simulink model "eVTOL_System"  (R2024b)
settings: Solver=FixedStepAuto  StartTime=0.0  StopTime=inf  RelTol=1e-3
undefined symbols (not defined in the file): airspeed, Battery, BCE12, BCE_Set_init, BMS_Controller_State, C, Cell10_P, Cell11_P, Cell12_P, Cell13_P, Cell14_P, Cell15_P, Cell16_P, Cell17_P, Cell18_P, Cell19_P, Cell1_N, Cell1_P, Cell20_P, Cell21_P, Cell22_P, Cell23_P, Cell24_P, Cell2_P, Cell3_P, Cell4_P, Cell5_P, Cell6_P, Cell7_P, Cell8_P, Cell9_P, Charging_State, CityMission, control, controlParams, ControlSampleTime, CriticalTiltAngle, currentFactor, CV_Gain, ddx, ddy, ddz, Device_01, Device_02, DiscIntNeverNeededParam, dx, dy, dz, Earth, env, F, F28379D_ADC_MaxCount, F28379D_ADC_Vmax, FixedWingMission, flightState, Foc_Ki_IxTcpu, Foc_Ki_S, Foc_Kp_I, Foc_Kp_S, fractalcoef ... (+68)
libraries: fl_lib x1115, nesl_utility x617, slrealtimeethercatlib x217, simulink x130, canmsglib x101, speedgoatlib_IO611_obsolete x91, slpidlib x49, mcbcontrolslib x44, slrealtimeutilitieslib x35, speedgoatlib_hdlCoder_IO3xx x31, dspstat3 x24, mcbpositiondecoderlib x12
(part 27 of 31)

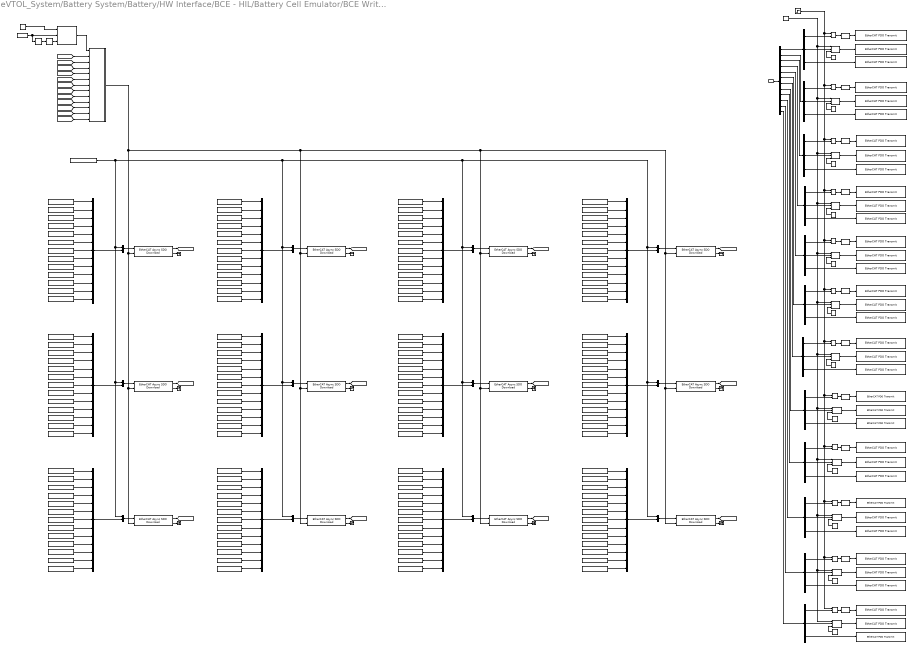
== system eVTOL_System/Battery System/Battery/HW Interface/BCE - HIL/Battery Cell Emulator/BCE Write 1/Subsystem/BCE Write  ==
  note: Task Scheduling
  note: Cell 4
  note: Cell 5
  note: Setup
  note: Cell 8
  note: Cell 8
  note: Cell 9
  note: Cell 1
  note: Cell 7
  note: Update
  note: Cell 2
  note: Cell 10
  note: Cell 1
  note: Cell 5
  note: Cell 3
  note: Cell 11
  note: Cell 10
  note: Cell 6
  note: Cell 7
  note: Cell 12
  note: Cell 6
  note: Cell 9
  note: Cell 11
  note: Cell 3
  note: Cell 12
  note: Cell 4
  note: Cell 2
  Data : Inport  OutDataTypeStr=Bus: BCE_Set
  BceVoltageLimit : Constant  Value=5  SampleTime=0.001
  Bus Selector : BusSelector  OutputSignals=Cell_1,Cell_2,Cell_3,Cell_4,Cell_5,Cell_6,Cell_7,Cell_8,Cell_9,Cell_10,Cell_11,Cell_12
  Bus Selector{1..12} (12 alike) : BusSelector  OutputSignals=Enable,V,I
  CellEnableDelay : Step  Time=2  SampleTime=0.001
  Constant{,1..11} (12 alike) : Constant  Value=0
  Data Type Conversion{1..12} (12 alike) : DataTypeConversion  OutDataTypeStr=uint8  SaturateOnIntegerOverflow=off  RndMeth=Floor
  Enable until confirmed : Subsystem
  EtherCAT Async SDO Download01 : slrealtimeethercatlib/EtherCAT Async SDO Download  index=0x4001  subIndex=1  sig_type=uint16  sig_dim=14  device_id=0  subdevice_name=Device_02 (BCE12-0505)  sample_time=0.001  subdevice_addr=1002  selected_subdevice=BCE_01  timeout=500  subdevice_found=0  complete=1
  EtherCAT Async SDO Download02 : slrealtimeethercatlib/EtherCAT Async SDO Download  index=0x4002  subIndex=1  sig_type=uint16  sig_dim=14  device_id=0  subdevice_name=Device_02 (BCE12-0505)  sample_time=0.001  subdevice_addr=1002  selected_subdevice=BCE_01  timeout=500  subdevice_found=0  complete=1
  EtherCAT Async SDO Download03 : slrealtimeethercatlib/EtherCAT Async SDO Download  index=0x4003  subIndex=1  sig_type=uint16  sig_dim=14  device_id=0  subdevice_name=Device_02 (BCE12-0505)  sample_time=0.001  subdevice_addr=1002  selected_subdevice=BCE_01  timeout=500  subdevice_found=0  complete=1
  EtherCAT Async SDO Download04 : slrealtimeethercatlib/EtherCAT Async SDO Download  index=0x4004  subIndex=1  sig_type=uint16  sig_dim=14  device_id=0  subdevice_name=Device_02 (BCE12-0505)  sample_time=0.001  subdevice_addr=1002  selected_subdevice=BCE_01  timeout=500  subdevice_found=0  complete=1
  EtherCAT Async SDO Download05 : slrealtimeethercatlib/EtherCAT Async SDO Download  index=0x4005  subIndex=1  sig_type=uint16  sig_dim=14  device_id=0  subdevice_name=Device_02 (BCE12-0505)  sample_time=0.001  subdevice_addr=1002  selected_subdevice=BCE_01  timeout=500  subdevice_found=0  complete=1
  EtherCAT Async SDO Download06 : slrealtimeethercatlib/EtherCAT Async SDO Download  index=0x4006  subIndex=1  sig_type=uint16  sig_dim=14  device_id=0  subdevice_name=Device_02 (BCE12-0505)  sample_time=0.001  subdevice_addr=1002  selected_subdevice=BCE_01  timeout=500  subdevice_found=0  complete=1
  EtherCAT Async SDO Download07 : slrealtimeethercatlib/EtherCAT Async SDO Download  index=0x4007  subIndex=0  sig_type=uint16  sig_dim=14  device_id=0  subdevice_name=Device_02 (BCE12-0505)  sample_time=0.001  subdevice_addr=1002  selected_subdevice=BCE_01  timeout=500  subdevice_found=0  complete=1
  EtherCAT Async SDO Download08 : slrealtimeethercatlib/EtherCAT Async SDO Download  index=0x4008  subIndex=0  sig_type=uint16  sig_dim=14  device_id=0  subdevice_name=Device_02 (BCE12-0505)  sample_time=0.001  subdevice_addr=1002  selected_subdevice=BCE_01  timeout=500  subdevice_found=0  complete=1
  EtherCAT Async SDO Download09 : slrealtimeethercatlib/EtherCAT Async SDO Download  index=0x4009  subIndex=1  sig_type=uint16  sig_dim=14  device_id=0  subdevice_name=Device_02 (BCE12-0505)  sample_time=0.001  subdevice_addr=1002  selected_subdevice=BCE_01  timeout=500  subdevice_found=0  complete=1
  EtherCAT Async SDO Download10 : slrealtimeethercatlib/EtherCAT Async SDO Download  index=0x400A  subIndex=1  sig_type=uint16  sig_dim=14  device_id=0  subdevice_name=Device_02 (BCE12-0505)  sample_time=0.001  subdevice_addr=1002  selected_subdevice=BCE_01  timeout=500  subdevice_found=0  complete=1
  EtherCAT Async SDO Download11 : slrealtimeethercatlib/EtherCAT Async SDO Download  index=0x400B  subIndex=1  sig_type=uint16  sig_dim=14  device_id=0  subdevice_name=Device_02 (BCE12-0505)  sample_time=0.001  subdevice_addr=1002  selected_subdevice=BCE_01  timeout=500  subdevice_found=0  complete=1
  EtherCAT Async SDO Download12 : slrealtimeethercatlib/EtherCAT Async SDO Download  index=0x400C  subIndex=1  sig_type=uint16  sig_dim=14  device_id=0  subdevice_name=Device_02 (BCE12-0505)  sample_time=0.001  subdevice_addr=1002  selected_subdevice=BCE_01  timeout=500  subdevice_found=0  complete=1
  EtherCAT PDO Transmit01 : slrealtimeethercatlib/EtherCAT PDO Transmit  Priority=3  sig_name=Device_02 (BCE12-0505).Rx_Cell_01.setVoltage  sig_offset=872  sig_type=single  type_size=32  sig_dim=1  device_id=0  sample_time=0.001000
  EtherCAT PDO Transmit02 : slrealtimeethercatlib/EtherCAT PDO Transmit  Priority=3  sig_name=Device_02 (BCE12-0505).Rx_Cell_01.setCurrent  sig_offset=904  sig_type=single  type_size=32  sig_dim=1  device_id=0  sample_time=0.001000
  EtherCAT PDO Transmit03 : slrealtimeethercatlib/EtherCAT PDO Transmit  Priority=3  sig_name=Device_02 (BCE12-0505).Rx_Cell_02.setVoltage  sig_offset=944  sig_type=single  type_size=32  sig_dim=1  device_id=0  sample_time=0.001000
  EtherCAT PDO Transmit04 : slrealtimeethercatlib/EtherCAT PDO Transmit  Priority=3  sig_name=Device_02 (BCE12-0505).Rx_Cell_02.setCurrent  sig_offset=976  sig_type=single  type_size=32  sig_dim=1  device_id=0  sample_time=0.001000
  EtherCAT PDO Transmit05 : slrealtimeethercatlib/EtherCAT PDO Transmit  Priority=3  sig_name=Device_02 (BCE12-0505).Rx_Cell_03.setVoltage  sig_offset=1016  sig_type=single  type_size=32  sig_dim=1  device_id=0  sample_time=0.001000
  EtherCAT PDO Transmit06 : slrealtimeethercatlib/EtherCAT PDO Transmit  Priority=3  sig_name=Device_02 (BCE12-0505).Rx_Cell_03.setCurrent  sig_offset=1048  sig_type=single  type_size=32  sig_dim=1  device_id=0  sample_time=0.001000
  EtherCAT PDO Transmit07 : slrealtimeethercatlib/EtherCAT PDO Transmit  Priority=3  sig_name=Device_02 (BCE12-0505).Rx_Cell_04.setVoltage  sig_offset=1088  sig_type=single  type_size=32  sig_dim=1  device_id=0  sample_time=0.001000
  EtherCAT PDO Transmit08 : slrealtimeethercatlib/EtherCAT PDO Transmit  Priority=3  sig_name=Device_02 (BCE12-0505).Rx_Cell_04.setCurrent  sig_offset=1120  sig_type=single  type_size=32  sig_dim=1  device_id=0  sample_time=0.001000
  EtherCAT PDO Transmit09 : slrealtimeethercatlib/EtherCAT PDO Transmit  Priority=3  sig_name=Device_02 (BCE12-0505).Rx_Cell_05.setVoltage  sig_offset=1160  sig_type=single  type_size=32  sig_dim=1  device_id=0  sample_time=0.001000
  EtherCAT PDO Transmit1 : slrealtimeethercatlib/EtherCAT PDO Transmit  Priority=3  sig_name=Device_02 (BCE12-0505).Rx_Cell_01.enableCell  sig_offset=864  sig_type=uint8  type_size=8  sig_dim=1  device_id=0  sample_time=0.001000
  EtherCAT PDO Transmit10 : slrealtimeethercatlib/EtherCAT PDO Transmit  Priority=3  sig_name=Device_02 (BCE12-0505).Rx_Cell_05.setCurrent  sig_offset=1192  sig_type=single  type_size=32  sig_dim=1  device_id=0  sample_time=0.001000
  EtherCAT PDO Transmit11 : slrealtimeethercatlib/EtherCAT PDO Transmit  Priority=3  sig_name=Device_02 (BCE12-0505).Rx_Cell_06.setVoltage  sig_offset=1232  sig_type=single  type_size=32  sig_dim=1  device_id=0  sample_time=0.001000
  EtherCAT PDO Transmit12 : slrealtimeethercatlib/EtherCAT PDO Transmit  Priority=3  sig_name=Device_02 (BCE12-0505).Rx_Cell_06.setCurrent  sig_offset=1264  sig_type=single  type_size=32  sig_dim=1  device_id=0  sample_time=0.001000
  EtherCAT PDO Transmit13 : slrealtimeethercatlib/EtherCAT PDO Transmit  Priority=3  sig_name=Device_02 (BCE12-0505).Rx_Cell_07.setVoltage  sig_offset=1304  sig_type=single  type_size=32  sig_dim=1  device_id=0  sample_time=0.001000
  EtherCAT PDO Transmit14 : slrealtimeethercatlib/EtherCAT PDO Transmit  Priority=3  sig_name=Device_02 (BCE12-0505).Rx_Cell_07.setCurrent  sig_offset=1336  sig_type=single  type_size=32  sig_dim=1  device_id=0  sample_time=0.001000
  EtherCAT PDO Transmit15 : slrealtimeethercatlib/EtherCAT PDO Transmit  Priority=3  sig_name=Device_02 (BCE12-0505).Rx_Cell_08.setVoltage  sig_offset=1376  sig_type=single  type_size=32  sig_dim=1  device_id=0  sample_time=0.001000
  EtherCAT PDO Transmit16 : slrealtimeethercatlib/EtherCAT PDO Transmit  Priority=3  sig_name=Device_02 (BCE12-0505).Rx_Cell_08.setCurrent  sig_offset=1408  sig_type=single  type_size=32  sig_dim=1  device_id=0  sample_time=0.001000
  EtherCAT PDO Transmit17 : slrealtimeethercatlib/EtherCAT PDO Transmit  Priority=3  sig_name=Device_02 (BCE12-0505).Rx_Cell_09.setVoltage  sig_offset=1448  sig_type=single  type_size=32  sig_dim=1  device_id=0  sample_time=0.001000
  EtherCAT PDO Transmit18 : slrealtimeethercatlib/EtherCAT PDO Transmit  Priority=3  sig_name=Device_02 (BCE12-0505).Rx_Cell_09.setCurrent  sig_offset=1480  sig_type=single  type_size=32  sig_dim=1  device_id=0  sample_time=0.001000
  EtherCAT PDO Transmit19 : slrealtimeethercatlib/EtherCAT PDO Transmit  Priority=3  sig_name=Device_02 (BCE12-0505).Rx_Cell_10.setVoltage  sig_offset=1520  sig_type=single  type_size=32  sig_dim=1  device_id=0  sample_time=0.001000
  EtherCAT PDO Transmit2 : slrealtimeethercatlib/EtherCAT PDO Transmit  Priority=3  sig_name=Device_02 (BCE12-0505).Rx_Cell_02.enableCell  sig_offset=936  sig_type=uint8  type_size=8  sig_dim=1  device_id=0  sample_time=0.001000
  EtherCAT PDO Transmit20 : slrealtimeethercatlib/EtherCAT PDO Transmit  Priority=3  sig_name=Device_02 (BCE12-0505).Rx_Cell_10.setCurrent  sig_offset=1552  sig_type=single  type_size=32  sig_dim=1  device_id=0  sample_time=0.001000
  EtherCAT PDO Transmit21 : slrealtimeethercatlib/EtherCAT PDO Transmit  Priority=3  sig_name=Device_02 (BCE12-0505).Rx_Cell_11.setVoltage  sig_offset=1592  sig_type=single  type_size=32  sig_dim=1  device_id=0  sample_time=0.001000
  EtherCAT PDO Transmit22 : slrealtimeethercatlib/EtherCAT PDO Transmit  Priority=3  sig_name=Device_02 (BCE12-0505).Rx_Cell_11.setCurrent  sig_offset=1624  sig_type=single  type_size=32  sig_dim=1  device_id=0  sample_time=0.001000
  EtherCAT PDO Transmit23 : slrealtimeethercatlib/EtherCAT PDO Transmit  Priority=3  sig_name=Device_02 (BCE12-0505).Rx_Cell_12.setVoltage  sig_offset=1664  sig_type=single  type_size=32  sig_dim=1  device_id=0  sample_time=0.001000
  EtherCAT PDO Transmit24 : slrealtimeethercatlib/EtherCAT PDO Transmit  Priority=3  sig_name=Device_02 (BCE12-0505).Rx_Cell_12.setCurrent  sig_offset=1696  sig_type=single  type_size=32  sig_dim=1  device_id=0  sample_time=0.001000
  EtherCAT PDO Transmit25 : slrealtimeethercatlib/EtherCAT PDO Transmit  Priority=3  sig_name=Device_02 (BCE12-0505).Rx_Cell_10.enableCell  sig_offset=1512  sig_type=uint8  type_size=8  sig_dim=1  device_id=0  sample_time=0.001000
  EtherCAT PDO Transmit26 : slrealtimeethercatlib/EtherCAT PDO Transmit  Priority=3  sig_name=Device_02 (BCE12-0505).Rx_Cell_11.enableCell  sig_offset=1584  sig_type=uint8  type_size=8  sig_dim=1  device_id=0  sample_time=0.001000
  EtherCAT PDO Transmit27 : slrealtimeethercatlib/EtherCAT PDO Transmit  Priority=3  sig_name=Device_02 (BCE12-0505).Rx_Cell_12.enableCell  sig_offset=1656  sig_type=uint8  type_size=8  sig_dim=1  device_id=0  sample_time=0.001000
  EtherCAT PDO Transmit3 : slrealtimeethercatlib/EtherCAT PDO Transmit  Priority=3  sig_name=Device_02 (BCE12-0505).Rx_Cell_03.enableCell  sig_offset=1008  sig_type=uint8  type_size=8  sig_dim=1  device_id=0  sample_time=0.001000
  EtherCAT PDO Transmit4 : slrealtimeethercatlib/EtherCAT PDO Transmit  Priority=3  sig_name=Device_02 (BCE12-0505).Rx_Cell_04.enableCell  sig_offset=1080  sig_type=uint8  type_size=8  sig_dim=1  device_id=0  sample_time=0.001000
  EtherCAT PDO Transmit5 : slrealtimeethercatlib/EtherCAT PDO Transmit  Priority=3  sig_name=Device_02 (BCE12-0505).Rx_Cell_05.enableCell  sig_offset=1152  sig_type=uint8  type_size=8  sig_dim=1  device_id=0  sample_time=0.001000
  EtherCAT PDO Transmit6 : slrealtimeethercatlib/EtherCAT PDO Transmit  Priority=3  sig_name=Device_02 (BCE12-0505).Rx_Cell_06.enableCell  sig_offset=1224  sig_type=uint8  type_size=8  sig_dim=1  device_id=0  sample_time=0.001000
  EtherCAT PDO Transmit7 : slrealtimeethercatlib/EtherCAT PDO Transmit  Priority=3  sig_name=Device_02 (BCE12-0505).Rx_Cell_07.enableCell  sig_offset=1296  sig_type=uint8  type_size=8  sig_dim=1  device_id=0  sample_time=0.001000
  EtherCAT PDO Transmit8 : slrealtimeethercatlib/EtherCAT PDO Transmit  Priority=3  sig_name=Device_02 (BCE12-0505).Rx_Cell_08.enableCell  sig_offset=1368  sig_type=uint8  type_size=8  sig_dim=1  device_id=0  sample_time=0.001000
  EtherCAT PDO Transmit9 : slrealtimeethercatlib/EtherCAT PDO Transmit  Priority=3  sig_name=Device_02 (BCE12-0505).Rx_Cell_09.enableCell  sig_offset=1440  sig_type=uint8  type_size=8  sig_dim=1  device_id=0  sample_time=0.001000
  EthercatNodeId : Constant  Value=2
  Logical Operator{,1..11} (12 alike) : Logic  AllPortsSameDT=off  OutDataTypeStr=boolean
  MATLAB Function : MATLAB Function  TreatAsAtomicUnit=on
  Mux{,1..11} (12 alike) : Mux  Inputs=13
  Mux{13..24} (12 alike) : Mux  Inputs=2
  NumElements : Constant  Value=14  OutDataTypeStr=uint16
  Probe : Probe  ProbeWidth=off  ProbeComplexSignal=off
  Saturation Dynamic{,1..11} (12 alike) : simulink/Discontinuities/Saturation Dynamic  OutMin=[]  OutMax=[]  OutDataTypeStr=Inherit: Same as second input  OutDataType=fixdt(1, 16)  OutScaling=2^-10  DoSatur=off
  Selector : Selector  InputPortWidth=2  IndexOptions=Index vector (dialog)  Indices=[1]  OutputSizes=1
  SimTime : DigitalClock  SampleTime=0.001
  Terminator{1,3,5,7,9,11,13,15,17,19,25,29} (12 alike) : Terminator
  advancedConfigRegisterCell{1..12} (12 alike) : Constant  Value=22658  OutDataTypeStr=uint16
  configRegisterCell{1..12} (12 alike) : Constant  Value=4370  OutDataTypeStr=uint16
  currentSinkLimitRegisterLsbCell{1..12} (12 alike) : Constant  Value=0  OutDataTypeStr=uint16
  currentSinkLimitRegisterMsbCell{1..12} (12 alike) : Constant  Value=0  OutDataTypeStr=uint16
  currentSourceLimitRegisterLsbCell{1..12} (12 alike) : Constant  Value=0  OutDataTypeStr=uint16
  currentSourceLimitRegisterMsbCell{1..12} (12 alike) : Constant  Value=0  OutDataTypeStr=uint16
  shutdownRegisterCell{1..12} (12 alike) : Constant  Value=31  OutDataTypeStr=uint16
  tempLowerLimitRegisterCell{1..12} (12 alike) : Constant  Value=65496  OutDataTypeStr=uint16
  tempUpperLimitRegisterCell{1..12} (12 alike) : Constant  Value=21760  OutDataTypeStr=uint16
  voltageLowerLimitRegisterLsbCell{1..12} (12 alike) : Constant  Value=0  OutDataTypeStr=uint16
  voltageLowerLimitRegisterMsbCell{1..12} (12 alike) : Constant  Value=0  OutDataTypeStr=uint16
  voltageUpperLimitRegisterLsbCell{1..12} (12 alike) : Constant  Value=0  OutDataTypeStr=uint16
  voltageUpperLimitRegisterMsbCell{1..12} (12 alike) : Constant  Value=0  OutDataTypeStr=uint16
  wires:
  Logical Operator11/1 -> Data Type Conversion12/1
  Logical Operator10/1 -> Data Type Conversion11/1
  Logical Operator9/1 -> Data Type Conversion10/1
  Logical Operator8/1 -> Data Type Conversion9/1
  Logical Operator7/1 -> Data Type Conversion8/1
  Logical Operator6/1 -> Data Type Conversion7/1
  Logical Operator5/1 -> Data Type Conversion6/1
  Logical Operator4/1 -> Data Type Conversion5/1
  Logical Operator3/1 -> Data Type Conversion4/1
  Logical Operator2/1 -> Data Type Conversion3/1
  Logical Operator1/1 -> Data Type Conversion2/1
  Logical Operator/1 -> Data Type Conversion1/1
  CellEnableDelay/1 -> Logical Operator/1, Logical Operator1/1, Logical Operator2/1, Logical Operator3/1, Logical Operator4/1, Logical Operator5/1, Logical Operator6/1, Logical Operator7/1, Logical Operator8/1, Logical Operator9/1, Logical Operator10/1, Logical Operator11/1
  Saturation Dynamic11/1 -> EtherCAT PDO Transmit23/1
  Constant11/1 -> Saturation Dynamic11/3
  Saturation Dynamic10/1 -> EtherCAT PDO Transmit21/1
  Constant10/1 -> Saturation Dynamic10/3
  Saturation Dynamic9/1 -> EtherCAT PDO Transmit19/1
  Constant9/1 -> Saturation Dynamic9/3
  Saturation Dynamic8/1 -> EtherCAT PDO Transmit17/1
  Constant8/1 -> Saturation Dynamic8/3
  Saturation Dynamic7/1 -> EtherCAT PDO Transmit15/1
  Constant7/1 -> Saturation Dynamic7/3
  Saturation Dynamic6/1 -> EtherCAT PDO Transmit13/1
  Constant6/1 -> Saturation Dynamic6/3
  Saturation Dynamic5/1 -> EtherCAT PDO Transmit11/1
  Constant5/1 -> Saturation Dynamic5/3
  Saturation Dynamic4/1 -> EtherCAT PDO Transmit09/1
  Constant4/1 -> Saturation Dynamic4/3
  Saturation Dynamic3/1 -> EtherCAT PDO Transmit07/1
  Constant3/1 -> Saturation Dynamic3/3
  Saturation Dynamic2/1 -> EtherCAT PDO Transmit05/1
  Constant2/1 -> Saturation Dynamic2/3
  Saturation Dynamic1/1 -> EtherCAT PDO Transmit03/1
  Constant1/1 -> Saturation Dynamic1/3
  BceVoltageLimit/1 -> Saturation Dynamic1/1, Saturation Dynamic2/1, Saturation Dynamic3/1, Saturation Dynamic4/1, Saturation Dynamic5/1, Saturation Dynamic6/1, Saturation Dynamic7/1, Saturation Dynamic8/1, Saturation Dynamic9/1, Saturation Dynamic10/1, Saturation Dynamic11/1, Saturation Dynamic/1
  Constant/1 -> Saturation Dynamic/3
  Saturation Dynamic/1 -> EtherCAT PDO Transmit01/1
  [cell12_download] -> Enable until confirmed/13(D12)
  [cell11_download] -> Enable until confirmed/12(D11)
  [cell10_download] -> Enable until confirmed/11(D10)
  [cell9_download] -> Enable until confirmed/10(D9)
  [cell8_download] -> Enable until confirmed/9(D8)
  [cell7_download] -> Enable until confirmed/8(D7)
  [cell6_download] -> Enable until confirmed/7(D6)
  [cell5_download] -> Enable until confirmed/6(D5)
  [cell4_download] -> Enable until confirmed/5(D4)
  [cell3_download] -> Enable until confirmed/4(D3)
  [cell2_download] -> Enable until confirmed/3(D2)
  [cell1_download] -> Enable until confirmed/2(D1)
  MATLAB Function/1(enable) -> Enable until confirmed/1(global enable)  "enable"
  currentSinkLimitRegisterLsbCell8/1 -> Mux7/10
  EtherCAT Async SDO Download08/2 -> Terminator29/1
  advancedConfigRegisterCell9/1 -> Mux8/3
  currentSourceLimitRegisterMsbCell2/1 -> Mux1/9
  Bus Selector6/3 -> EtherCAT PDO Transmit12/1  "<I>"
  currentSinkLimitRegisterMsbCell5/1 -> Mux4/11
  Bus Selector/4 -> Bus Selector4/1  "<Cell_4>"
  voltageUpperLimitRegisterLsbCell1/1 -> Mux/4
  currentSinkLimitRegisterLsbCell11/1 -> Mux10/10
  Mux10/1 -> Mux22/2
  currentSourceLimitRegisterLsbCell8/1 -> Mux7/8
  currentSinkLimitRegisterMsbCell12/1 -> Mux11/11
  EtherCAT Async SDO Download01/2 -> Terminator1/1
  Data Type Conversion7/1 -> EtherCAT PDO Transmit7/1
  EtherCAT Async SDO Download12/2 -> Terminator19/1
  Bus Selector11/3 -> EtherCAT PDO Transmit22/1  "<I>"
  EtherCAT Async SDO Download04/2 -> Terminator7/1
  shutdownRegisterCell10/1 -> Mux9/2
  Enable until confirmed/1(Out1) -> EtherCAT Async SDO Download12/2, EtherCAT Async SDO Download11/2, EtherCAT Async SDO Download10/2, EtherCAT Async SDO Download09/2, EtherCAT Async SDO Download08/2, EtherCAT Async SDO Download07/2, EtherCAT Async SDO Download06/2, EtherCAT Async SDO Download05/2, EtherCAT Async SDO Download04/2, EtherCAT Async SDO Download03/2, EtherCAT Async SDO Download02/2, EtherCAT Async SDO Download01/2
  tempUpperLimitRegisterCell6/1 -> Mux5/12
  Bus Selector9/3 -> EtherCAT PDO Transmit18/1  "<I>"
  Bus Selector/8 -> Bus Selector8/1  "<Cell_8>"
  tempLowerLimitRegisterCell9/1 -> Mux8/13
  EtherCAT Async SDO Download12/1 -> [cell12_download]
  voltageLowerLimitRegisterLsbCell4/1 -> Mux3/6
  Bus Selector8/2 -> Saturation Dynamic7/2  "<V>"
  advancedConfigRegisterCell8/1 -> Mux7/3
  currentSourceLimitRegisterLsbCell5/1 -> Mux4/8
  voltageLowerLimitRegisterLsbCell2/1 -> Mux1/6
  Bus Selector12/1 -> Logical Operator11/2  "<Enable>"
  Bus Selector5/2 -> Saturation Dynamic4/2  "<V>"
  voltageUpperLimitRegisterLsbCell2/1 -> Mux1/4
  Bus Selector8/1 -> Logical Operator7/2  "<Enable>"
  currentSinkLimitRegisterLsbCell10/1 -> Mux9/10
  shutdownRegisterCell6/1 -> Mux5/2
  voltageLowerLimitRegisterMsbCell12/1 -> Mux11/7
  Mux17/1 -> EtherCAT Async SDO Download06/1
  Mux13/1 -> EtherCAT Async SDO Download02/1
  voltageLowerLimitRegisterMsbCell3/1 -> Mux2/7
  advancedConfigRegisterCell5/1 -> Mux4/3
  shutdownRegisterCell1/1 -> Mux/2
  shutdownRegisterCell5/1 -> Mux4/2
  Data Type Conversion11/1 -> EtherCAT PDO Transmit26/1
  Mux20/1 -> EtherCAT Async SDO Download09/1
  tempLowerLimitRegisterCell1/1 -> Mux/13
  voltageUpperLimitRegisterMsbCell6/1 -> Mux5/5
  Bus Selector1/1 -> Logical Operator/2  "<Enable>"
  Bus Selector5/3 -> EtherCAT PDO Transmit10/1  "<I>"
  Data/1 -> Bus Selector/1
  tempUpperLimitRegisterCell4/1 -> Mux3/12
  tempLowerLimitRegisterCell10/1 -> Mux9/13
  Mux15/1 -> EtherCAT Async SDO Download04/1
  EtherCAT Async SDO Download09/1 -> [cell9_download]
  voltageUpperLimitRegisterLsbCell8/1 -> Mux7/4
  tempUpperLimitRegisterCell3/1 -> Mux2/12
  currentSinkLimitRegisterLsbCell9/1 -> Mux8/10
  Mux14/1 -> EtherCAT Async SDO Download03/1
  Bus Selector10/3 -> EtherCAT PDO Transmit20/1  "<I>"
  tempUpperLimitRegisterCell10/1 -> Mux9/12
  advancedConfigRegisterCell12/1 -> Mux11/3
  advancedConfigRegisterCell2/1 -> Mux1/3
  tempLowerLimitRegisterCell12/1 -> Mux11/13
  currentSinkLimitRegisterMsbCell11/1 -> Mux10/11
  voltageUpperLimitRegisterMsbCell7/1 -> Mux6/5
  voltageUpperLimitRegisterLsbCell3/1 -> Mux2/4
  currentSourceLimitRegisterMsbCell7/1 -> Mux6/9
  currentSourceLimitRegisterLsbCell12/1 -> Mux11/8
  voltageLowerLimitRegisterMsbCell2/1 -> Mux1/7
  currentSourceLimitRegisterLsbCell7/1 -> Mux6/8
  Bus Selector/11 -> Bus Selector11/1  "<Cell_11>"
  voltageLowerLimitRegisterLsbCell6/1 -> Mux5/6
  tempUpperLimitRegisterCell12/1 -> Mux11/12
  Bus Selector3/2 -> Saturation Dynamic2/2  "<V>"
  voltageUpperLimitRegisterMsbCell8/1 -> Mux7/5
  voltageUpperLimitRegisterMsbCell1/1 -> Mux/5
  shutdownRegisterCell9/1 -> Mux8/2
  voltageUpperLimitRegisterLsbCell4/1 -> Mux3/4
  Bus Selector2/3 -> EtherCAT PDO Transmit04/1  "<I>"
  currentSourceLimitRegisterMsbCell12/1 -> Mux11/9
  currentSourceLimitRegisterMsbCell5/1 -> Mux4/9
  tempLowerLimitRegisterCell2/1 -> Mux1/13
  EtherCAT Async SDO Download10/2 -> Terminator15/1
  currentSourceLimitRegisterMsbCell10/1 -> Mux9/9
  Bus Selector5/1 -> Logical Operator4/2  "<Enable>"
  tempUpperLimitRegisterCell1/1 -> Mux/12
  currentSourceLimitRegisterLsbCell11/1 -> Mux10/8
  voltageLowerLimitRegisterLsbCell11/1 -> Mux10/6
  Bus Selector10/2 -> Saturation Dynamic9/2  "<V>"
  EtherCAT Async SDO Download06/2 -> Terminator11/1
  currentSourceLimitRegisterMsbCell6/1 -> Mux5/9
  Bus Selector12/3 -> EtherCAT PDO Transmit24/1  "<I>"
  Selector/1 -> MATLAB Function/3(Ts)
  Bus Selector/5 -> Bus Selector5/1  "<Cell_5>"
  voltageUpperLimitRegisterMsbCell9/1 -> Mux8/5
  Bus Selector/10 -> Bus Selector10/1  "<Cell_10>"
  Bus Selector1/3 -> EtherCAT PDO Transmit02/1  "<I>"
  voltageLowerLimitRegisterMsbCell4/1 -> Mux3/7
  Data Type Conversion3/1 -> EtherCAT PDO Transmit3/1
  voltageUpperLimitRegisterMsbCell2/1 -> Mux1/5
  tempUpperLimitRegisterCell5/1 -> Mux4/12
  currentSinkLimitRegisterMsbCell7/1 -> Mux6/11
  shutdownRegisterCell2/1 -> Mux1/2
  currentSourceLimitRegisterMsbCell4/1 -> Mux3/9
  EtherCAT Async SDO Download05/1 -> [cell5_download]
  Bus Selector4/1 -> Logical Operator3/2  "<Enable>"
  EtherCAT Async SDO Download11/1 -> [cell11_download]
  currentSinkLimitRegisterLsbCell4/1 -> Mux3/10
  currentSinkLimitRegisterLsbCell2/1 -> Mux1/10
  tempLowerLimitRegisterCell7/1 -> Mux6/13
  Mux24/1 -> EtherCAT Async SDO Download01/1
  voltageUpperLimitRegisterLsbCell10/1 -> Mux9/4
  currentSourceLimitRegisterLsbCell2/1 -> Mux1/8
  Bus Selector4/2 -> Saturation Dynamic3/2  "<V>"
  tempLowerLimitRegisterCell5/1 -> Mux4/13
  configRegisterCell9/1 -> Mux8/1
  advancedConfigRegisterCell6/1 -> Mux5/3
  Bus Selector6/2 -> Saturation Dynamic5/2  "<V>"
  Bus Selector3/3 -> EtherCAT PDO Transmit06/1  "<I>"
  voltageLowerLimitRegisterLsbCell8/1 -> Mux7/6
  Mux4/1 -> Mux16/2
  voltageLowerLimitRegisterLsbCell9/1 -> Mux8/6
  Bus Selector/12 -> Bus Selector12/1  "<Cell_12>"
  voltageUpperLimitRegisterMsbCell11/1 -> Mux10/5
  Bus Selector4/3 -> EtherCAT PDO Transmit08/1  "<I>"
  currentSinkLimitRegisterMsbCell1/1 -> Mux/11
  voltageLowerLimitRegisterMsbCell11/1 -> Mux10/7
  advancedConfigRegisterCell3/1 -> Mux2/3
  currentSinkLimitRegisterMsbCell2/1 -> Mux1/11
  configRegisterCell1/1 -> Mux/1
  advancedConfigRegisterCell4/1 -> Mux3/3
  voltageLowerLimitRegisterLsbCell1/1 -> Mux/6
  currentSourceLimitRegisterMsbCell9/1 -> Mux8/9
  currentSourceLimitRegisterMsbCell3/1 -> Mux2/9
  Data Type Conversion1/1 -> EtherCAT PDO Transmit1/1
  Mux/1 -> Mux24/2  "MUX_OUTPUT"
  Data Type Conversion10/1 -> EtherCAT PDO Transmit25/1
  tempUpperLimitRegisterCell7/1 -> Mux6/12
  Data Type Conversion12/1 -> EtherCAT PDO Transmit27/1
  Data Type Conversion5/1 -> EtherCAT PDO Transmit5/1
  Data Type Conversion9/1 -> EtherCAT PDO Transmit9/1
  Data Type Conversion6/1 -> EtherCAT PDO Transmit6/1
  currentSinkLimitRegisterMsbCell9/1 -> Mux8/11
  currentSinkLimitRegisterLsbCell3/1 -> Mux2/10
  Data Type Conversion4/1 -> EtherCAT PDO Transmit4/1
  currentSourceLimitRegisterMsbCell11/1 -> Mux10/9
  EtherCAT Async SDO Download01/1 -> [cell1_download]
  configRegisterCell2/1 -> Mux1/1
  EtherCAT Async SDO Download02/2 -> Terminator3/1
  tempUpperLimitRegisterCell11/1 -> Mux10/12
  EtherCAT Async SDO Download10/1 -> [cell10_download]
  Bus Selector/9 -> Bus Selector9/1  "<Cell_9>"
  Bus Selector7/3 -> EtherCAT PDO Transmit14/1  "<I>"
  advancedConfigRegisterCell10/1 -> Mux9/3
  Mux11/1 -> Mux23/2
  configRegisterCell3/1 -> Mux2/1
  voltageUpperLimitRegisterMsbCell12/1 -> Mux11/5
  voltageUpperLimitRegisterMsbCell4/1 -> Mux3/5
  currentSourceLimitRegisterLsbCell1/1 -> Mux/8
  Bus Selector7/2 -> Saturation Dynamic6/2  "<V>"
  Mux6/1 -> Mux18/2
  configRegisterCell10/1 -> Mux9/1
  currentSinkLimitRegisterMsbCell3/1 -> Mux2/11
  Data Type Conversion2/1 -> EtherCAT PDO Transmit2/1
  configRegisterCell11/1 -> Mux10/1
  Bus Selector/6 -> Bus Selector6/1  "<Cell_6>"
  Bus Selector/2 -> Bus Selector2/1  "<Cell_2>"
  tempLowerLimitRegisterCell3/1 -> Mux2/13
  Bus Selector1/2 -> Saturation Dynamic/2  "<V>"
  advancedConfigRegisterCell11/1 -> Mux10/3
  Mux22/1 -> EtherCAT Async SDO Download11/1
  Mux18/1 -> EtherCAT Async SDO Download07/1
  Bus Selector11/1 -> Logical Operator10/2  "<Enable>"
  configRegisterCell5/1 -> Mux4/1
  voltageUpperLimitRegisterMsbCell3/1 -> Mux2/5
  Bus Selector/3 -> Bus Selector3/1  "<Cell_3>"
  voltageLowerLimitRegisterMsbCell10/1 -> Mux9/7
  tempLowerLimitRegisterCell6/1 -> Mux5/13
  Mux8/1 -> Mux20/2
  Bus Selector8/3 -> EtherCAT PDO Transmit16/1  "<I>"
  tempLowerLimitRegisterCell11/1 -> Mux10/13
  Mux9/1 -> Mux21/2
  voltageLowerLimitRegisterLsbCell5/1 -> Mux4/6
  Bus Selector/1 -> Bus Selector1/1  "<Cell_1>"
  EthercatNodeId/1 -> MATLAB Function/1(nodeNbr)
  EtherCAT Async SDO Download03/1 -> [cell3_download]
  Bus Selector11/2 -> Saturation Dynamic10/2  "<V>"
  Bus Selector/7 -> Bus Selector7/1  "<Cell_7>"
  tempUpperLimitRegisterCell2/1 -> Mux1/12
  voltageLowerLimitRegisterMsbCell5/1 -> Mux4/7
  Probe/1 -> Selector/1
  EtherCAT Async SDO Download02/1 -> [cell2_download]
  currentSourceLimitRegisterLsbCell6/1 -> Mux5/8
  tempLowerLimitRegisterCell4/1 -> Mux3/13
  voltageUpperLimitRegisterMsbCell10/1 -> Mux9/5
  currentSinkLimitRegisterMsbCell8/1 -> Mux7/11
  configRegisterCell7/1 -> Mux6/1
  voltageUpperLimitRegisterMsbCell5/1 -> Mux4/5
  currentSourceLimitRegisterLsbCell10/1 -> Mux9/8
  EtherCAT Async SDO Download09/2 -> Terminator13/1
  shutdownRegisterCell12/1 -> Mux11/2
  NumElements/1 -> Mux23/1, Mux22/1, Mux21/1, Mux20/1, Mux19/1, Mux18/1, Mux17/1, Mux16/1, Mux15/1, Mux14/1, Mux13/1, Mux24/1
  currentSourceLimitRegisterLsbCell4/1 -> Mux3/8
  configRegisterCell6/1 -> Mux5/1
  shutdownRegisterCell3/1 -> Mux2/2
  shutdownRegisterCell8/1 -> Mux7/2
  currentSinkLimitRegisterLsbCell1/1 -> Mux/10
  Bus Selector3/1 -> Logical Operator2/2  "<Enable>"
  voltageUpperLimitRegisterLsbCell7/1 -> Mux6/4
  Bus Selector2/1 -> Logical Operator1/2  "<Enable>"
  Bus Selector10/1 -> Logical Operator9/2  "<Enable>"
  voltageUpperLimitRegisterLsbCell11/1 -> Mux10/4
  Bus Selector2/2 -> Saturation Dynamic1/2  "<V>"
  configRegisterCell12/1 -> Mux11/1
  voltageLowerLimitRegisterMsbCell1/1 -> Mux/7
  EtherCAT Async SDO Download03/2 -> Terminator5/1
  SimTime/1 -> Probe/1, MATLAB Function/2(simTime)
  voltageLowerLimitRegisterLsbCell3/1 -> Mux2/6
  voltageUpperLimitRegisterLsbCell5/1 -> Mux4/4
  EtherCAT Async SDO Download07/1 -> [cell7_download]
  advancedConfigRegisterCell7/1 -> Mux6/3
  currentSourceLimitRegisterMsbCell8/1 -> Mux7/9
  voltageUpperLimitRegisterLsbCell12/1 -> Mux11/4
  currentSourceLimitRegisterLsbCell9/1 -> Mux8/8
  Mux7/1 -> Mux19/2
  tempUpperLimitRegisterCell8/1 -> Mux7/12
  currentSinkLimitRegisterMsbCell6/1 -> Mux5/11
  Bus Selector9/1 -> Logical Operator8/2  "<Enable>"
  Mux23/1 -> EtherCAT Async SDO Download12/1
  Mux16/1 -> EtherCAT Async SDO Download05/1
  Bus Selector12/2 -> Saturation Dynamic11/2  "<V>"
  configRegisterCell4/1 -> Mux3/1
  voltageLowerLimitRegisterLsbCell7/1 -> Mux6/6
  voltageUpperLimitRegisterLsbCell9/1 -> Mux8/4
  Mux3/1 -> Mux15/2
  voltageLowerLimitRegisterLsbCell12/1 -> Mux11/6
  Mux1/1 -> Mux13/2
  voltageLowerLimitRegisterLsbCell10/1 -> Mux9/6
  Bus Selector9/2 -> Saturation Dynamic8/2  "<V>"
  EtherCAT Async SDO Download04/1 -> [cell4_download]
  shutdownRegisterCell11/1 -> Mux10/2
  currentSourceLimitRegisterLsbCell3/1 -> Mux2/8
  currentSinkLimitRegisterLsbCell5/1 -> Mux4/10
  EtherCAT Async SDO Download11/2 -> Terminator17/1
  EtherCAT Async SDO Download08/1 -> [cell8_download]
  EtherCAT Async SDO Download07/2 -> Terminator25/1
  shutdownRegisterCell4/1 -> Mux3/2
  Mux5/1 -> Mux17/2
  currentSinkLimitRegisterMsbCell10/1 -> Mux9/11
  EtherCAT Async SDO Download06/1 -> [cell6_download]
  Mux19/1 -> EtherCAT Async SDO Download08/1
  advancedConfigRegisterCell1/1 -> Mux/3
  tempLowerLimitRegisterCell8/1 -> Mux7/13
  Mux2/1 -> Mux14/2
  voltageLowerLimitRegisterMsbCell7/1 -> Mux6/7
  currentSinkLimitRegisterLsbCell12/1 -> Mux11/10
  Mux21/1 -> EtherCAT Async SDO Download10/1
  voltageUpperLimitRegisterLsbCell6/1 -> Mux5/4
  currentSinkLimitRegisterLsbCell6/1 -> Mux5/10
  Data Type Conversion8/1 -> EtherCAT PDO Transmit8/1
  currentSinkLimitRegisterLsbCell7/1 -> Mux6/10
  voltageLowerLimitRegisterMsbCell8/1 -> Mux7/7
  EtherCAT Async SDO Download05/2 -> Terminator9/1
  Bus Selector7/1 -> Logical Operator6/2  "<Enable>"
  voltageLowerLimitRegisterMsbCell9/1 -> Mux8/7
  configRegisterCell8/1 -> Mux7/1
  shutdownRegisterCell7/1 -> Mux6/2
  Bus Selector6/1 -> Logical Operator5/2  "<Enable>"
  voltageLowerLimitRegisterMsbCell6/1 -> Mux5/7
  currentSinkLimitRegisterMsbCell4/1 -> Mux3/11
  tempUpperLimitRegisterCell9/1 -> Mux8/12
  currentSourceLimitRegisterMsbCell1/1 -> Mux/9

== system eVTOL_System/Dynamics/Force and Moments/Aerodynamic Forces/Compute Body Frame Forces and Moments/Wind frame F& M/Lateral Channel/CY/roll factors ==
  p,q,r : Inport
  Airspeed : Inport  Port=2
  Constant : Constant  Value=uavParam.aero.CYp
      settings: AttributesFormatString=%<Value>
  Constant1 : Constant  Value=uavParam.aero.CYr
      settings: AttributesFormatString=%<Value>
  Get p : Selector  InputPortWidth=3  IndexOptions=Index vector (dialog)  Indices=1  OutputSizes=[(-2)]
  Get r : Selector  InputPortWidth=3  IndexOptions=Index vector (dialog)  Indices=3  OutputSizes=[(-2)]
  Product : Product  SaturateOnIntegerOverflow=on  OutDataTypeStr=Inherit: Same as first input
  Product1 : Product  SaturateOnIntegerOverflow=on  OutDataTypeStr=Inherit: Same as first input
  Subsystem : Subsystem
  roll rate fact : Subsystem
  CYp : Outport  VectorParamsAs1DForOutWhenUnconnected=off
  CYr : Outport  Port=2  VectorParamsAs1DForOutWhenUnconnected=off
  wires:
  Get r/1 -> Subsystem/1(r)
  p,q,r/1 -> Get r/1, Get p/1
  Get p/1 -> roll rate fact/1(p)
  Airspeed/1 -> Subsystem/2(Airspeed), roll rate fact/2(Airspeed)
  Subsystem/1(Yaw Rate Fac) -> Product1/2
  Constant1/1 -> Product1/1
  roll rate fact/1(Roll Rate Fac) -> Product/2
  Constant/1 -> Product/1
  Product1/1 -> CYr/1
  Product/1 -> CYp/1

== system eVTOL_System/Dynamics/Force and Moments/Aerodynamic Forces/Compute Body Frame Forces and Moments/Wind frame F& M/Lateral Channel/Cl/roll factors ==
  p,q,r : Inport
  Airspeed : Inport  Port=2
  Constant : Constant  Value=uavParam.aero.Clp
      settings: AttributesFormatString=%<Value>
  Constant1 : Constant  Value=uavParam.aero.Clr
      settings: AttributesFormatString=%<Value>
  Get p : Selector  InputPortWidth=3  IndexOptions=Index vector (dialog)  Indices=1  OutputSizes=[(-2)]
  Get r : Selector  InputPortWidth=3  IndexOptions=Index vector (dialog)  Indices=3  OutputSizes=[(-2)]
  Product : Product  SaturateOnIntegerOverflow=on  OutDataTypeStr=Inherit: Same as first input
  Product1 : Product  SaturateOnIntegerOverflow=on  OutDataTypeStr=Inherit: Same as first input
  roll rate fact : Subsystem
  yaw rate fact : mbdriLib/Utilities/yaw rate fact  SystemSampleTime=-1  VariantActivationTime=update diagram  AllowFlexibleInterface=on  Latency=0  AutoFrameSizeCalculation=off
      link override Cmq4: Value=uavParam.geom.b
  Clp : Outport  VectorParamsAs1DForOutWhenUnconnected=off
  Clr : Outport  Port=2  VectorParamsAs1DForOutWhenUnconnected=off
  wires:
  Get r/1 -> yaw rate fact/1
  p,q,r/1 -> Get r/1, Get p/1
  Get p/1 -> roll rate fact/1(p)
  Airspeed/1 -> yaw rate fact/2, roll rate fact/2(Airspeed)
  yaw rate fact/1 -> Product1/2
  Constant1/1 -> Product1/1
  roll rate fact/1(Roll Rate Fac) -> Product/2
  Constant/1 -> Product/1
  Product1/1 -> Clr/1
  Product/1 -> Clp/1

== system eVTOL_System/Dynamics/Force and Moments/Aerodynamic Forces/Compute Body Frame Forces and Moments/Wind frame F& M/Lateral Channel/Cn/yaw factors ==
  p,q,r : Inport
  Airspeed : Inport  Port=2
  Constant : Constant  Value=uavParam.aero.Cnp
      settings: AttributesFormatString=%<Value>
  Constant1 : Constant  Value=uavParam.aero.Cnr
      settings: AttributesFormatString=%<Value>
  Get p : Selector  InputPortWidth=3  IndexOptions=Index vector (dialog)  Indices=1  OutputSizes=[(-2)]
  Get r : Selector  InputPortWidth=3  IndexOptions=Index vector (dialog)  Indices=3  OutputSizes=[(-2)]
  Product : Product  SaturateOnIntegerOverflow=on  OutDataTypeStr=Inherit: Same as first input
  Product1 : Product  SaturateOnIntegerOverflow=on  OutDataTypeStr=Inherit: Same as first input
  roll rate fact : Subsystem
  yaw rate fact : mbdriLib/Utilities/yaw rate fact  SystemSampleTime=-1  VariantActivationTime=update diagram  AllowFlexibleInterface=on  Latency=0  AutoFrameSizeCalculation=off
      link override Cmq4: Value=uavParam.geom.b
  Cnp : Outport  VectorParamsAs1DForOutWhenUnconnected=off
  Cnr : Outport  Port=2  VectorParamsAs1DForOutWhenUnconnected=off
  wires:
  Airspeed/1 -> yaw rate fact/2, roll rate fact/2(Airspeed)
  Get r/1 -> yaw rate fact/1
  p,q,r/1 -> Get r/1, Get p/1
  Get p/1 -> roll rate fact/1(p)
  roll rate fact/1(Roll Rate Fac) -> Product/2
  Constant/1 -> Product/1
  yaw rate fact/1 -> Product1/2
  Constant1/1 -> Product1/1
  Product1/1 -> Cnr/1
  Product/1 -> Cnp/1

== system eVTOL_System/Dynamics/Force and Moments/Aerodynamic Forces/Compute Body Frame Forces and Moments/Wind frame F& M/Longitudinal Channel/CL/Lift due to pitch rate ==
  p,q,r : Inport
  Airspeed : Inport  Port=2
  Constant : Constant  Value=uavParam.aero.CLq
      settings: AttributesFormatString=%<Value>
  Get q : Selector  InputPortWidth=3  IndexOptions=Index vector (dialog)  Indices=2  OutputSizes=[(-2)]
  Product : Product  SaturateOnIntegerOverflow=on  OutDataTypeStr=Inherit: Same as first input
  pitch rate factor : Subsystem
  CLq : Outport  VectorParamsAs1DForOutWhenUnconnected=off
  wires:
  Airspeed/1 -> pitch rate factor/2(Airspeed)
  Get q/1 -> pitch rate factor/1(q)
  p,q,r/1 -> Get q/1
  Product/1 -> CLq/1
  pitch rate factor/1(Pitch Rate Fac) -> Product/2
  Constant/1 -> Product/1

== system eVTOL_System/Dynamics/Force and Moments/Aerodynamic Forces/Compute Body Frame Forces and Moments/Wind frame F& M/Longitudinal Channel/Cm/Lift due to pitch rate ==
  p,q,r : Inport
  Airspeed : Inport  Port=2
  Constant : Constant  Value=uavParam.aero.Cmq
      settings: AttributesFormatString=%<Value>
  Get q : Selector  InputPortWidth=3  IndexOptions=Index vector (dialog)  Indices=2  OutputSizes=[(-2)]
  Product : Product  SaturateOnIntegerOverflow=on  OutDataTypeStr=Inherit: Same as first input
  pitch rate factor : Subsystem
  Cmq : Outport  VectorParamsAs1DForOutWhenUnconnected=off
  wires:
  Airspeed/1 -> pitch rate factor/2(Airspeed)
  Get q/1 -> pitch rate factor/1(q)
  p,q,r/1 -> Get q/1
  Product/1 -> Cmq/1
  pitch rate factor/1(Pitch Rate Fac) -> Product/2
  Constant/1 -> Product/1

== system eVTOL_System/Flight Controller/Guidance Test Bench/ControlType/Guidance Testbench/Guidance Logic/Guidance Stateflow/Guidance Mode Selector/GuidanceLogic.WP/Back Transition Guard ==
  note: Set previous waypoint to current location if the UAV has just exited back transition
  Poses : Inport
  FromWP : Inport  Port=2
  Bus Selector : BusSelector  OutputSignals=mode
  Bus Selector1 : BusSelector  OutputSignals=position,params,mode
  Constant : Constant  Value=6
  Equal : RelationalOperator  Operator===  OutDataTypeStr=boolean  RndMeth=Simplest  InputSameDT=off
  Switch : Switch  Criteria=u2 > Threshold  SaturateOnIntegerOverflow=off  InputSameDT=off
  Triggered Subsystem : Subsystem  TreatAsAtomicUnit=on
  Out Bus Element2 : Outport  PortName=PrevWP  Element=mode
  Out Bus Element : Outport  PortName=PrevWP  Element=position
  Out Bus Element1 : Outport  PortName=PrevWP  Element=params
  wires:
  FromWP/1 -> Bus Selector1/1, Bus Selector/1
  Bus Selector/1 -> Equal/2  "<mode>"
  Constant/1 -> Equal/1
  Equal/1 -> Switch/2, Triggered Subsystem/Trigger
  Poses/1 -> Triggered Subsystem/1(Poses)
  Triggered Subsystem/1(HoldPositionValue) -> Switch/1
  Bus Selector1/1 -> Switch/3  "<position>"
  Switch/1 -> Out Bus Element/1
  Bus Selector1/2 -> Out Bus Element1/1  "<params>"
  Bus Selector1/3 -> Out Bus Element2/1  "<mode>"

== system eVTOL_System/Flight Controller/Guidance Test Bench/ControlType/Guidance Testbench/Guidance Logic/Guidance Stateflow/Guidance Mode Selector/GuidanceLogic.WP/Dist2WP ==
  Pose : Inport
  FromWP : Inport  Port=2
  ToWP : Inport  Port=3
  Bus Selector : BusSelector  OutputSignals=position
  Bus Selector1 : BusSelector  OutputSignals=position
  Demux : Demux  Outputs=[3 1]
  Dot Product : DotProduct  OutDataTypeStr=Inherit: Inherit via internal rule
  Subsystem : Subsystem
  Sum : Sum  Inputs=|-+
  Sum1 : Sum  Inputs=|+-
  Terminator : Terminator
  Dist : Outport
  wires:
  Sum1/1 -> Subsystem/1(V)
  Demux/2 -> Terminator/1
  Bus Selector/1 -> Sum/2, Sum1/1  "<position>"
  Demux/1 -> Sum/1
  Bus Selector1/1 -> Sum1/2  "<position>"
  Sum/1 -> Dot Product/1
  Subsystem/1(V_unit) -> Dot Product/2
  Pose/1 -> Demux/1
  Dot Product/1 -> Dist/1
  ToWP/1 -> Bus Selector/1
  FromWP/1 -> Bus Selector1/1

== system eVTOL_System/Motor Drive/Controller/Controller_MIL/F28379D Firmware/Controller Algorithm/FOC/Current Control/Control_System ==
  Iab_meas_PU : Inport
  Pos_PU : Inport  Port=2
  Enable : Inport  Port=3
  Idq_ref_PU : Inport  Port=4
  SpeedRef : Inport  Port=5
  Kp_i : Inport  Port=6
  Ki_ixTcpu : Inport  Port=7
  Closed Loop Control : Subsystem
  Demux : Demux  Outputs=2
  NOT : Logic  Operator=NOT  IconShape=distinctive  AllPortsSameDT=off  OutDataTypeStr=boolean
  Open Loop Start-Up : Subsystem
  Output Scaling : Subsystem
  Switch : Switch  Criteria=u2 > Threshold  Threshold=0.5  SaturateOnIntegerOverflow=off  InputSameDT=off
  ModWave : Outport
  PWM_Enable : Outport  Port=2
  Idq_debug : Outport  Port=3  VectorParamsAs1DForOutWhenUnconnected=off
  wires:
  Open Loop Start-Up/1(PWM_Duty) -> Switch/3
  Switch/1 -> Output Scaling/1(PWM_Duty)
  Enable/1 -> Demux/1
  Demux/1 -> Closed Loop Control/Enable, Switch/2, NOT/1
  Demux/2 -> [EnablePWM], Open Loop Start-Up/1(<EnablePWM>)
  Iab_meas_PU/1 -> Closed Loop Control/1(Iab_meas_PU)
  Pos_PU/1 -> Closed Loop Control/2(Pos_PU)
  Idq_ref_PU/1 -> Closed Loop Control/3(Idq_ref_PU)  "idqref"
  [EnablePWM] -> Closed Loop Control/4(EnablePWM)
  Closed Loop Control/1(Idq_debug) -> Idq_debug/1
  Closed Loop Control/2(Vabc in PU) -> Switch/1
  Output Scaling/1(ModWave) -> ModWave/1
  Output Scaling/2(PWM_Enable) -> PWM_Enable/1
  [EnablePWM] -> Output Scaling/2(Enable)
  SpeedRef/1 -> Open Loop Start-Up/2(SpeedRef)
  NOT/1 -> Open Loop Start-Up/Enable
  Ki_ixTcpu/1 -> Closed Loop Control/6(Ki_ixTcpu)
  Kp_i/1 -> Closed Loop Control/5(Kp_i)

== system eVTOL_System/Motor Drive/Controller/Controller_MIL/F28379D Firmware/Controller Algorithm/FOC/Speed Control MLD/PI_Controller_Speed ==
  Enable : Inport
  N_ref : Inport  Port=2
  N_fb : Inport  Port=3
  Kp_S : Inport  Port=4
  Ki_S : Inport  Port=5
  Discrete PI Controller with anti-windup & reset : slpidlib/PID Controller  Controller=PI  Form=Parallel  TimeDomain=Discrete-time  UseExternalTs=off  SampleTime=-1  IntegratorMethod=Forward Euler  FilterMethod=Forward Euler  ControllerParametersSource=external  P=1  I=1  UseKiTs=on  D=0  UseExternalDerivativeSource=off  N=100  UseFilter=on  TunerSelectOption=Transfer Function Based (PID Tuner App)  InitialConditionSource=external  InitialConditionForIntegrator=0  InitialConditionForFilter=0  DifferentiatorICPrevScaledInput=0  ExternalReset=level  TrackingMode=off  Kt=1  LimitOutput=on  SatLimitsSource=internal  UpperSaturationLimit=1  LowerSaturationLimit=-1  LinearizeAsGain=on  AntiWindupMode=clamping  Kb=1  LimitIntegrator=off  UpperIntegratorSaturationLimit=inf  LowerIntegratorSaturationLimit=-inf  RndMeth=Simplest  POutMin=[]  POutMax=[]  IOutMin=[]  IOutMax=[]  DOutMin=[]  DOutMax=[]  NOutMin=[]  NOutMax=[]  SumOutMin=[]  SumOutMax=[]  SaturationOutDataTypeStr=Inherit: Inherit via back propagation  SaturationOutMin=[]  SaturationOutMax=[]  PParamMin=[]  PParamMax=[]  IParamMin=[]  IParamMax=[]  DParamMin=[]  DParamMax=[]  NParamMin=[]  NParamMax=[]  KbParamMin=[]  KbParamMax=[]  KtParamMin=[]  KtParamMax=[]  KbOutMin=[]  KbOutMax=[]  KtOutMin=[]  KtOutMax=[]  IntegratorOutMin=[]  IntegratorOutMax=[]  FilterOutMin=[]  FilterOutMax=[]  SumI1OutMin=[]  SumI1OutMax=[]  SumI2OutMin=[]  SumI2OutMax=[]  SumI3OutMin=[]  SumI3OutMax=[]  SumI4OutMin=[]  SumI4OutMax=[]  SumDOutMin=[]  SumDOutMax=[]  DifferentiatorOutMin=[]  DifferentiatorOutMax=[]  FilterDiffOutCoefMin=[]  FilterDiffOutCoefMax=[]  ReciprocalOutMin=[]  ReciprocalOutMax=[]  SumDenOutMin=[]  SumDenOutMax=[]  SumNumOutMin=[]  SumNumOutMax=[]  DivideOutMin=[]  DivideOutMax=[]  UdiffTsProdOutMin=[]  UdiffTsProdOutMax=[]  NTsProdOutMin=[]  NTsProdOutMax=[]  UintegralTsProdOutMin=[]  UintegralTsProdOutMax=[]  UngainTsProdOutMin=[]  UngainTsProdOutMax=[]  ClampingZeroOutDataTypeStr=Inherit: Inherit via back propagation  ClampingZeroOutMin=[]  ClampingZeroOutMax=[]  FilterDenConstantOutDataTypeStr=Inherit: Inherit via back propagation  FilterDenConstantOutMin=[]  FilterDenConstantOutMax=[]  PCopyOutDataTypeStr=Inherit: Inherit via back propagation  PCopyOutMin=[]  PCopyOutMax=[]  NCopyOutDataTypeStr=Inherit: Inherit via back propagation  NCopyOutMin=[]  NCopyOutMax=[]  IntegratorContinuousStateAttributes=''  IntegratorStateMustResolveToSignalObject=off  IntegratorRTWStateStorageClass=Auto  FilterContinuousStateAttributes=''  FilterStateMustResolveToSignalObject=off  FilterRTWStateStorageClass=Auto  ParallelPVariant=ExternalParameters  IdealPVariant=Disabled  IVariant=ExternalParameters  DVariant=Disabled  IntegratorVariant=Discrete  SatVariant=Enabled  AWVariant=DiscClampingParallel  PCopyVariant=Disabled  TRVariant=Disabled  FdbkBlocksVariant=Forward  IdealPFdbkVariant=Disabled  SatFdbkVariant=Disabled  DerivativeFilterVariant=Disabled  NVariant=Disabled  NCopyVariant=Disabled_SignalSpec  FilterICVariant=Disabled  IntegratorICVariant=ExternalICs  ExternalResetVariant=ExternalReset  TRSumVariant=Passthrough  SumFdbkVariant=Disabled  SumVariant=Sum_PI  TsampFilterVariant=InternalTs  TsampNgainVariant=Passthrough  TsampIntegralVariant=Disabled_SignalSpec  ExternalSaturationOutDataTypeStr=Inherit: Same as second input  DerivativeSourceVariant=Disabled  PreIntVariant=InternalPreInt
  Ki2 : Constant  Value=0  OutDataTypeStr=single  SampleTime=-1
  Logical Operator : Logic  Operator=NOT  IconShape=distinctive  AllPortsSameDT=off  OutDataTypeStr=boolean
  Sum : Sum  Inputs=|+-  OutDataTypeStr=Inherit: Same as first input
  Iq_ref : Outport  VectorParamsAs1DForOutWhenUnconnected=off
  wires:
  Ki_S/1 -> Discrete PI Controller with anti-windup & reset/3
  Kp_S/1 -> Discrete PI Controller with anti-windup & reset/2
  Enable/1 -> Logical Operator/1
  Ki2/1 -> Discrete PI Controller with anti-windup & reset/5
  Logical Operator/1 -> Discrete PI Controller with anti-windup & reset/4
  Sum/1 -> Discrete PI Controller with anti-windup & reset/1
  N_ref/1 -> Sum/1
  N_fb/1 -> Sum/2
  Discrete PI Controller with anti-windup & reset/1 -> Iq_ref/1

== system eVTOL_System/Motor Drive/Controller/Controller_MIL/F28379D Firmware/Controller Algorithm/FOC/Speed Control MLD/Speed_Ref_Selector ==
  Enable : Inport
  SpeedCommand : Inport  Port=2
  Speed_Ref_Open : Inport  Port=3
  IIR Filter : mcbcontrolslib/IIR Filter  VariantControl=Low Pass Filter  VariantSelect=Low-pass  FilterConstantInputType=Specify via dialog  Filter_constant=0.01  advancedSettings=off  Ts=50e-6  cutOff_freq=32.1525
  Switch : Switch  Criteria=u2 > Threshold  Threshold=0.5  SaturateOnIntegerOverflow=off  InputSameDT=off
  Speed_Ref_PU : Outport
  wires:
  SpeedCommand/1 -> Switch/1  "SpeedRef"
  Enable/1 -> Switch/2
  Speed_Ref_Open/1 -> Switch/3
  Switch/1 -> IIR Filter/1
  IIR Filter/1 -> Speed_Ref_PU/1

== system eVTOL_System/Motor Drive/Controller1/Controller_MIL/F28379D Firmware/Controller Algorithm/FOC/Current Control/Control_System ==
  Iab_meas_PU : Inport
  Pos_PU : Inport  Port=2
  Enable : Inport  Port=3
  Idq_ref_PU : Inport  Port=4
  SpeedRef : Inport  Port=5
  Kp_i : Inport  Port=6
  Ki_ixTcpu : Inport  Port=7
  Closed Loop Control : Subsystem
  Demux : Demux  Outputs=2
  NOT : Logic  Operator=NOT  IconShape=distinctive  AllPortsSameDT=off  OutDataTypeStr=boolean
  Open Loop Start-Up : Subsystem
  Output Scaling : Subsystem
  Switch : Switch  Criteria=u2 > Threshold  Threshold=0.5  SaturateOnIntegerOverflow=off  InputSameDT=off
  ModWave : Outport
  PWM_Enable : Outport  Port=2
  Idq_debug : Outport  Port=3  VectorParamsAs1DForOutWhenUnconnected=off
  wires:
  Open Loop Start-Up/1(PWM_Duty) -> Switch/3
  Switch/1 -> Output Scaling/1(PWM_Duty)
  Enable/1 -> Demux/1
  Demux/1 -> Closed Loop Control/Enable, Switch/2, NOT/1
  Demux/2 -> [EnablePWM], Open Loop Start-Up/1(<EnablePWM>)
  Iab_meas_PU/1 -> Closed Loop Control/1(Iab_meas_PU)
  Pos_PU/1 -> Closed Loop Control/2(Pos_PU)
  Idq_ref_PU/1 -> Closed Loop Control/3(Idq_ref_PU)  "idqref"
  [EnablePWM] -> Closed Loop Control/4(EnablePWM)
  Closed Loop Control/1(Idq_debug) -> Idq_debug/1
  Closed Loop Control/2(Vabc in PU) -> Switch/1
  Output Scaling/1(ModWave) -> ModWave/1
  Output Scaling/2(PWM_Enable) -> PWM_Enable/1
  [EnablePWM] -> Output Scaling/2(Enable)
  SpeedRef/1 -> Open Loop Start-Up/2(SpeedRef)
  NOT/1 -> Open Loop Start-Up/Enable
  Ki_ixTcpu/1 -> Closed Loop Control/6(Ki_ixTcpu)
  Kp_i/1 -> Closed Loop Control/5(Kp_i)
